simulink model "ntnu_leg"  (R2022b)
settings: Solver=VariableStepAuto  StartTime=0.0  StopTime=1  MaxStep=1e-3  RelTol=1e-3  AbsTol=1e-6
settings Model: Creator=papaveneti  LastModifiedBy=papaveneti

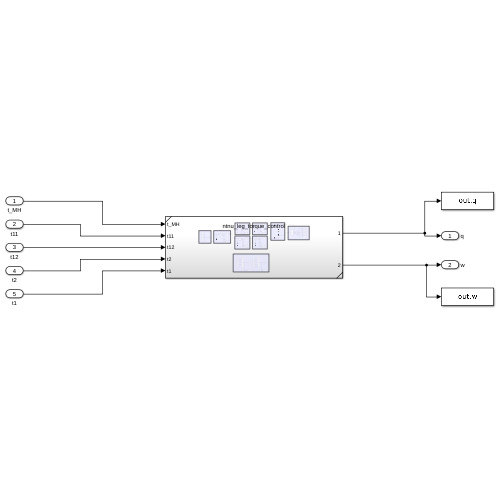
[thumbnail: Simulink's stored preview of the top-level diagram]
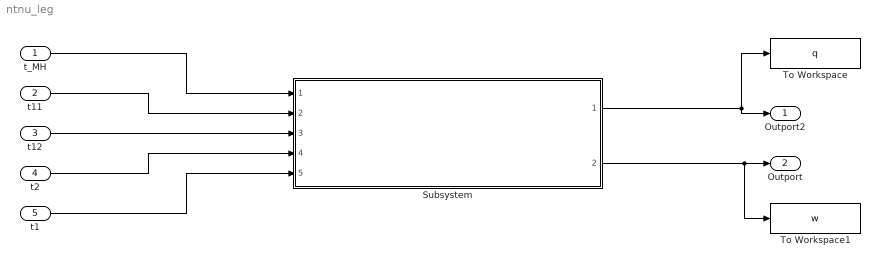
== system ntnu_leg ==
  t_MH : Inport
  t11 : Inport  Port=2
  t12 : Inport  Port=3
  t2 : Inport  Port=4
  t1 : Inport  Port=5
  Subsystem : Subsystem  ReferencedSubsystem=ntnu_leg_torque_control
  To Workspace : ToWorkspace  VariableName=q  SaveFormat=Timeseries  SampleTime=-1
  To Workspace1 : ToWorkspace  VariableName=w  SaveFormat=Timeseries  SampleTime=-1
  Outport2 : Outport  SignalName=q
  Outport : Outport  Port=2  SignalName=w
  wires:
  t_MH/1 -> Subsystem/1
  t11/1 -> Subsystem/2
  t12/1 -> Subsystem/3
  t2/1 -> Subsystem/4
  t1/1 -> Subsystem/5
  Subsystem/1 -> Outport2/1, To Workspace/1
  Subsystem/2 -> To Workspace1/1, Outport/1
